simulink model "MathModel_Boost_Subsys_ClosedLoop_org"  (Simulink 10.0)
settings: Solver=ode45  StartTime=0.0  StopTime=0.2  RelTol=1e-3  EnableMultiTasking=on
libraries: simulink x1, powerlib_meascontrol x1
settings Model: Creator=Landon  LastModifiedBy=annonymous
settings DataIOCC: LimitDataPoints=on
settings DebuggingCC: UnderspecifiedInitializationDetection=Simplified  MergeDetectMultiDrivingBlocksExec=error
settings GRTTargetCC: GeneratePreprocessorConditionals=Disable all  CombineOutputUpdateFcns=on  GRTInterface=off
settings ConfigComp: CovExternalEMLEnable=off

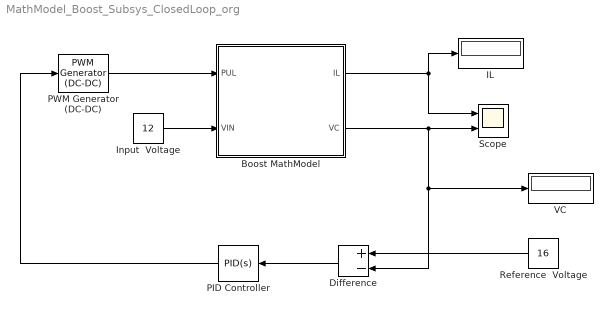
== system MathModel_Boost_Subsys_ClosedLoop_org ==
  Boost MathModel : Subsystem  mask{L=1.5e-3, C=250e-6, R=3}
      mask prompts: L "Inductance (H)"; C "Capacitance (F)"; R "Load Resistance (Ohm)"
  Difference : Sum  Inputs=+-
  IL : Display
  Input  Voltage : Constant  Value=12  VectorParams1D=off
  PID Controller : simulink/Continuous/PID Controller  Controller=PID  Form=Parallel  TimeDomain=Continuous-time  SampleTime=-1  IntegratorMethod=Forward Euler  FilterMethod=Forward Euler  ControllerParametersSource=internal  P=0  I=7.5  D=0  UseFilter=on  N=100  TunerSelectOption=Transfer Function Based (PID Tuner App)  InitialConditionSource=internal  InitialConditionForIntegrator=0  InitialConditionForFilter=0  DifferentiatorICPrevScaledInput=0  ExternalReset=none  TrackingMode=off  Kt=1  LimitOutput=off  UpperSaturationLimit=1e6  LowerSaturationLimit=-1e6  LinearizeAsGain=off  AntiWindupMode=none  Kb=1  POutMin=[]  POutMax=[]  IOutMin=[]  IOutMax=[]  DOutMin=[]  DOutMax=[]  NOutMin=[]  NOutMax=[]  SumOutMin=[]  SumOutMax=[]  SaturationOutMin=[]  SaturationOutMax=[]  PParamMin=[]  PParamMax=[]  IParamMin=[]  IParamMax=[]  DParamMin=[]  DParamMax=[]  NParamMin=[]  NParamMax=[]  KbParamMin=[]  KbParamMax=[]  KtParamMin=[]  KtParamMax=[]  KbOutMin=[]  KbOutMax=[]  KtOutMin=[]  KtOutMax=[]  IntegratorOutMin=[]  IntegratorOutMax=[]  FilterOutMin=[]  FilterOutMax=[]  SumI1OutMin=[]  SumI1OutMax=[]  SumI2OutMin=[]  SumI2OutMax=[]  SumI3OutMin=[]  SumI3OutMax=[]  SumI4OutMin=[]  SumI4OutMax=[]  SumDOutMin=[]  SumDOutMax=[]  DifferentiatorOutMin=[]  DifferentiatorOutMax=[]  FilterDiffOutCoefMin=[]  FilterDiffOutCoefMax=[]  ReciprocalOutMin=[]  ReciprocalOutMax=[]  SumDenOutMin=[]  SumDenOutMax=[]  SumNumOutMin=[]  SumNumOutMax=[]  DivideOutMin=[]  DivideOutMax=[]  IntegratorContinuousStateAttributes=''  IntegratorStateMustResolveToSignalObject=off  IntegratorRTWStateStorageClass=Auto  FilterContinuousStateAttributes=''  FilterStateMustResolveToSignalObject=off  FilterRTWStateStorageClass=Auto  ParallelPVariant=InternalParameters  IdealPVariant=Disabled  IVariant=InternalParameters  DVariant=InternalParameters  IntegratorVariant=Continuous  SatVariant=Disabled  AWVariant=Passthrough  PCopyVariant=Disabled  TRVariant=Disabled  FdbkBlocksVariant=Forward  IdealPFdbkVariant=Disabled  SatFdbkVariant=Disabled  DerivativeFilterVariant=ContFilter  NVariant=InternalParameters  NCopyVariant=Disabled  FilterICVariant=InternalICsFilter  IntegratorICVariant=InternalICs  ExternalResetVariant=Disabled  TRSumVariant=Passthrough  SumFdbkVariant=Disabled  SumVariant=Sum_PID
  PWM Generator (DC-DC) : powerlib_meascontrol/Pulse & Signal Generators/PWM Generator (DC-DC)  Fsw=5000  Ts=0
      settings: SourceProductName=Simscape Electrical
  Reference  Voltage : Constant  Value=16
  Scope : Scope  NumInputPorts=2
  VC : Display
  wires:
  Difference/1 -> PID Controller/1
  Reference  Voltage/1 -> Difference/1
  PID Controller/1 -> PWM Generator (DC-DC)/1
  Boost MathModel/1(IL) -> Scope/1, IL/1
  Boost MathModel/2(VC) -> Difference/2, VC/1, Scope/2
  PWM Generator (DC-DC)/1 -> Boost MathModel/1(PUL)
  Input  Voltage/1 -> Boost MathModel/2(VIN)

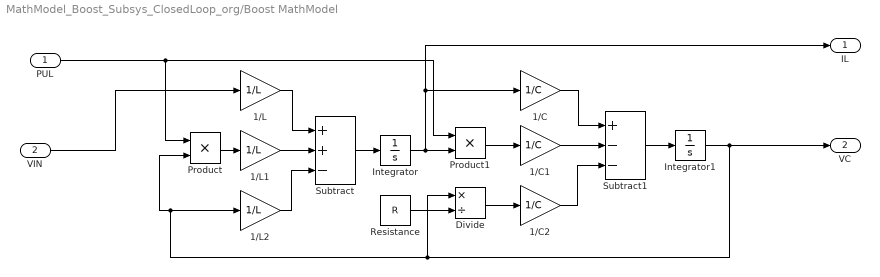
== system MathModel_Boost_Subsys_ClosedLoop_org/Boost MathModel ==
  PUL : Inport
  VIN : Inport  Port=2
  1/C : Gain  Gain=1/C
  1/C1 : Gain  Gain=1/C
  1/C2 : Gain  Gain=1/C
  1/L : Gain  Gain=1/L
  1/L1 : Gain  Gain=1/L
  1/L2 : Gain  Gain=1/L
  Divide : Product  Inputs=*/
  Integrator : Integrator
  Integrator1 : Integrator
  Product : Product
  Product1 : Product
  Resistance : Constant  Value=R
  Subtract : Sum  Inputs=++-
  Subtract1 : Sum  Inputs=+--
  IL : Outport
  VC : Outport  Port=2
  wires:
  1/C/1 -> Subtract1/1
  1/L1/1 -> Subtract/2
  Divide/1 -> 1/C2/1
  Product/1 -> 1/L1/1
  VIN/1 -> 1/L/1
  Subtract/1 -> Integrator/1
  Resistance/1 -> Divide/2
  1/L2/1 -> Subtract/3
  Integrator1/1 -> VC/1, 1/L2/1, Product/2, Divide/1
  Subtract1/1 -> Integrator1/1
  1/C2/1 -> Subtract1/3
  Integrator/1 -> Product1/2, IL/1, 1/C/1
  PUL/1 -> Product1/1, Product/1
  1/L/1 -> Subtract/1
  Product1/1 -> 1/C1/1
  1/C1/1 -> Subtract1/2
